simulink model "TP_Automatique_suspension_simulink"  (R2024a)
settings: Solver=ode45  StartTime=0.0  StopTime=10.0  RelTol=1e-3  EnableMultiTasking=on
values from neighbouring files (symbols this model uses):
  R = 24*10^3    (= 24000)    [TP Automatique.m]    (also in TP_Automatique.m = [r_0, r_1, r_2, r_3]; TP_Automatique_2.m = Vecteur_solution(4:7); TP_Automatique_suspension.m = [r_0, r_1, r_2, r_3]; chat.m = theta(1:nr+1).')
  S = [1, sigma_1, sigma_2, sigma_3]    [TP_Automatique.m]    (also in TP_Automatique_2.m = Vecteur_solution(1:3); TP_Automatique_suspension.m = [1, sigma_1, sigma_2, sigma_3, 0]; chat.m = [SA SB]; matlab.mat = [1 40.9 681.8 6077.6 0])
  T = 26.330 * [1 30 300 1000]    [TP_Automatique.m]    (also in TP_Automatique_2.m; TP_Automatique_suspension.m; chat.m = T(end-nb:end))
  U_0 = R*I_0    (= 15570018.9474)    [TP Automatique.m]    (also in TP_Automatique.m = R*I_0; TP_Automatique_2.m = R*I_0; TP_Automatique_suspension.m = R*I_0; chat.m = R*I_0)
  V = poly([-1 , -1, -1, -1])    [TP_Automatique.m]    (also in TP_Automatique_suspension.m; matlab.mat = [1 4 6 4 1])
  V_0 = -alpha*Z_0    (= -15)    [TP_Automatique.m]    (also in TP_Automatique_2.m; TP_Automatique_suspension.m; chat.m)
undefined symbols (not defined in the file or in its folder): sigbuilder_block
settings Model: Creator=2021-1254  LastModifiedBy=Administrator
settings SolverCC: AlgebraicLoopSolver=TrustRegion
settings DataIOCC: LimitDataPoints=on  SaveFormat=Array  ReturnWorkspaceOutputs=off
settings OptimizationCC: LifeSpan=inf
settings DebuggingCC: UnderspecifiedInitializationDetection=Classic  MergeDetectMultiDrivingBlocksExec=none  SolverPrmCheckMsg=warning  UnconnectedInputMsg=warning  UnconnectedOutputMsg=warning  UnconnectedLineMsg=warning  SFUnexpectedBacktrackingDiag=warning  SFNoUnconditionalDefaultTransitionDiag=warning  SFExecutionAtInitializationDiag=none  ArithmeticOperatorsInVariantConditions=warning
settings HardwareCC: ProdBitPerPointer=32  ProdBitPerSizeT=32  ProdBitPerPtrDiffT=32  ProdLargestAtomicFloat=None  ProdIntDivRoundTo=Undefined  ProdEndianess=Unspecified  ProdWordSize=32  ProdHWDeviceType=32-bit Generic
settings ModelReferenceCC: PropagateSignalLabelsOutOfModel=off
settings SFSimCC: SimUseLocalCustomCode=off  CustomCodeUndefinedFunction=UseInterfaceOnly
settings RTWCC: RTWUseLocalCustomCode=off  GPUComputeCapability=3.5
settings CodeAppCC: StateflowObjectComments=on
settings GRTTargetCC: TargetLangStandard=C89/C90 (ANSI)
settings ConfigComp: CovMetricSettings=dw  CovSaveCumulativeToWorkspaceVar=on  CovSaveSingleToWorkspaceVar=on  CovExternalEMLEnable=off

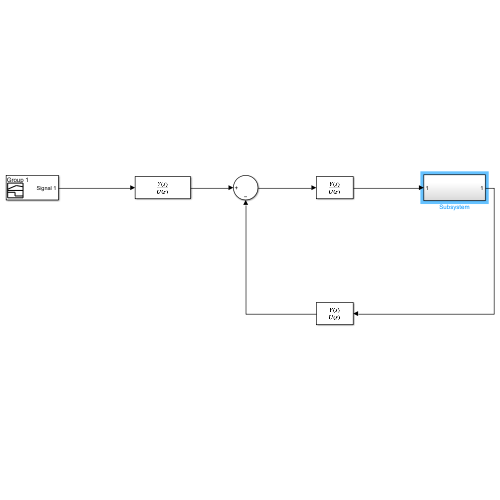
[thumbnail: Simulink's stored preview of the top-level diagram]
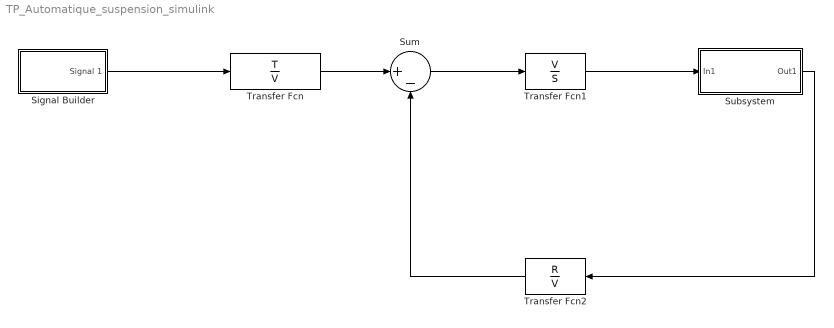
== system TP_Automatique_suspension_simulink ==
  Signal Builder : Subsystem  Tag=STV Subsys  LoadFcn=sigbuilder_block('load');  StartFcn=sigbuilder_block('start');  StopFcn=sigbuilder_block('stop');  ClipboardFcn=sigbuilder_block('clipboard');  mask(Sigbuilder block){tuvar=[0:10]}
      mask help: Simulink:masks:SigbuilderBlock_MD
      mask init:
      | if ~strcmp(get_param(bdroot(gcbh),'SimulationStatus'),'stopped') tuvar = sigbuilder_block('maskInit'); end
      settings: CopyFcn=sigbuilder_block('copy');  DeleteFcn=sigbuilder_block('delete');  ModelCloseFcn=sigbuilder_block('modelClose');  PreSaveFcn=sigbuilder_block('preSave');  PauseFcn=sigbuilder_block('pause');  ContinueFcn=sigbuilder_block('continue');  NameChangeFcn=sigbuilder_block('namechange');  OpenFcn=sigbuilder_block('open',[-284.25 -135 1428 717.75 ]);  CloseFcn=sigbuilder_block('close');
      mask Display: plot(0, 0, 100, 100,[2, 2, 32, 32, 2], [68, 8, 8, 68, 68],[32, 2], [38, 38], [32, 19, 2],[53, 60, 44], [32, 17, 17, 2],[16, 16, 31, 31]);txt = getActiveGroup(gcbh);text(2, 100, txt,'verticalAlignment', 'top');
  Subsystem : Subsystem
  Sum : Sum  Inputs=|+-
  Transfer Fcn : TransferFcn  Numerator=T  Denominator=V
  Transfer Fcn1 : TransferFcn  Numerator=V  Denominator=S
  Transfer Fcn2 : TransferFcn  Numerator=R  Denominator=V
  wires:
  Signal Builder/1(Signal 1) -> Transfer Fcn/1
  Transfer Fcn/1 -> Sum/1
  Transfer Fcn2/1 -> Sum/2
  Transfer Fcn1/1 -> Subsystem/1(In1)
  Sum/1 -> Transfer Fcn1/1
  Subsystem/1(Out1) -> Transfer Fcn2/1

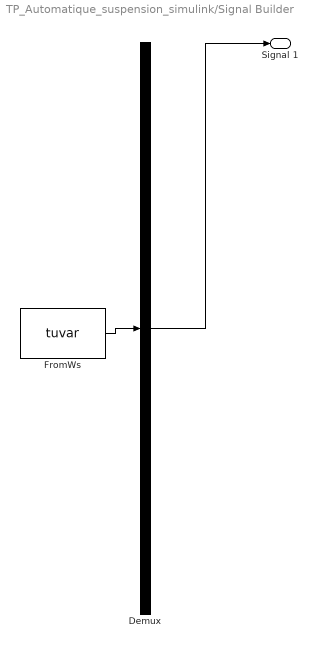
== system TP_Automatique_suspension_simulink/Signal Builder ==
  Demux : Demux  Tag=STV Demux  Outputs=1
      settings: DisplayOption=none
  FromWs : FromWorkspace  Tag=STV FromWs  VariableName=tuvar
      SigBuilderData=|
      | common.afterFinalStr = 'Extrapolate'
      | common.sampleTime = 0
      | dataSet.timeRange = [0 50]
      | dataSet.name = 'Group 1'
      | sbobj.Groups.Name = 'Group 1'
      | sbobj.Groups.Signals.Name = 'Signal 1'
      | sbobj.Groups.Signals.XData = [0 10 10 20 20 30 30 50]
      | sbobj.Groups.Signals.YData = [0 0 -10 -10 -20 -20 0 0]
      | sbobj.Groups.TimeRange = [0 50]
  Signal 1 : Outport  Tag=STV Outport
  wires:
  Demux/1 -> Signal 1/1
  FromWs/1 -> Demux/1

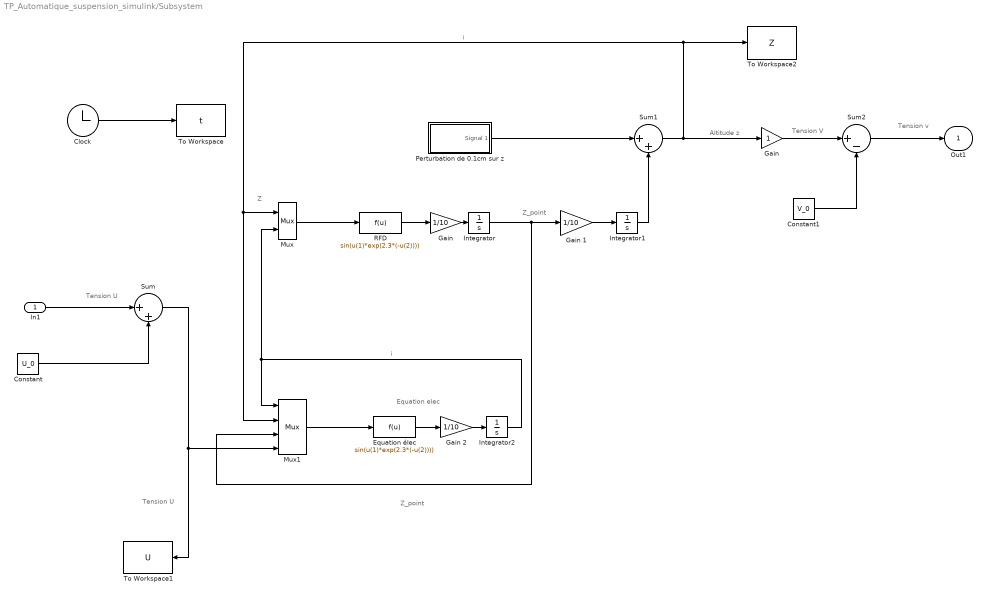
== system TP_Automatique_suspension_simulink/Subsystem ==
  note: Tension v
  note: Tension V
  note: Altitude z
  note: Z
  note: Z_point
  note: Equation elec
  note: Z_point
  note: Tension U
  note: Tension U
  In1 : Inport
  Clock : Clock
  Constant : Constant  Value=U_0
  Constant1 : Constant  Value=V_0
  Equation élec : Fcn  Expr=sin(u(1)*exp(2.3*(-u(2))))
  Gain : Gain
  "Gain " : Gain  Gain=1/10
  "Gain 1 " : Gain  Gain=1/10
  "Gain 2 " : Gain  Gain=1/10
  Integrator : Integrator
  Integrator1 : Integrator
  Integrator2 : Integrator
  Mux : Mux  Inputs=2
  Mux1 : Mux
  Perturbation de 0.1cm sur z : Subsystem  Tag=STV Subsys  LoadFcn=sigbuilder_block('load');  StartFcn=sigbuilder_block('start');  StopFcn=sigbuilder_block('stop');  ClipboardFcn=sigbuilder_block('clipboard');  mask(Sigbuilder block){tuvar=[0:10]}
      mask help: Simulink:masks:SigbuilderBlock_MD
      mask init:
      | if ~strcmp(get_param(bdroot(gcbh),'SimulationStatus'),'stopped') tuvar = sigbuilder_block('maskInit'); end
      settings: CopyFcn=sigbuilder_block('copy');  DeleteFcn=sigbuilder_block('delete');  ModelCloseFcn=sigbuilder_block('modelClose');  PreSaveFcn=sigbuilder_block('preSave');  PauseFcn=sigbuilder_block('pause');  ContinueFcn=sigbuilder_block('continue');  NameChangeFcn=sigbuilder_block('namechange');  OpenFcn=sigbuilder_block('open',[236 5.5 718.5 474.5 ]);  CloseFcn=sigbuilder_block('close');
      mask Display: plot(0, 0, 100, 100,[2, 2, 32, 32, 2], [68, 8, 8, 68, 68],[32, 2], [38, 38], [32, 19, 2],[53, 60, 44], [32, 17, 17, 2],[16, 16, 31, 31]);txt = getActiveGroup(gcbh);text(2, 100, txt,'verticalAlignment', 'top');
  RFD : Fcn  Expr=sin(u(1)*exp(2.3*(-u(2))))
  Sum : Sum  Inputs=|++
  Sum1 : Sum  Inputs=|++
  Sum2 : Sum  Inputs=|+-
  To Workspace : ToWorkspace  VariableName=t  SampleTime=-1
  To Workspace1 : ToWorkspace  VariableName=U  SampleTime=-1
  To Workspace2 : ToWorkspace  VariableName=Z  SampleTime=-1
  Out1 : Outport
  wires:
  In1/1 -> Sum/1
  Constant/1 -> Sum/2
  Clock/1 -> To Workspace/1
  Mux1/1 -> Equation élec/1
  Equation élec/1 -> "Gain 2 "/1
  Sum/1 -> To Workspace1/1, Mux1/4
  Mux/1 -> RFD/1
  RFD/1 -> "Gain "/1
  Perturbation de 0.1cm sur z/1(Signal 1) -> Sum1/1
  Gain/1 -> Sum2/1
  Sum2/1 -> Out1/1
  Integrator1/1 -> Sum1/2
  Integrator/1 -> Mux1/3, "Gain 1 "/1
  Constant1/1 -> Sum2/2
  Sum1/1 -> To Workspace2/1, Mux1/2, Mux/1, Gain/1  "i"
  Integrator2/1 -> Mux1/1, Mux/2  "i"
  "Gain "/1 -> Integrator/1
  "Gain 1 "/1 -> Integrator1/1
  "Gain 2 "/1 -> Integrator2/1

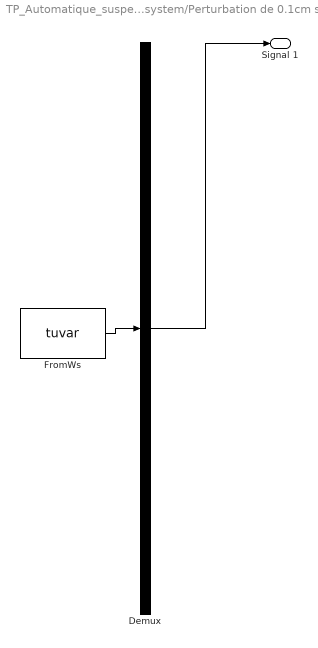
== system TP_Automatique_suspension_simulink/Subsystem/Perturbation de 0.1cm sur z ==
  Demux : Demux  Tag=STV Demux  Outputs=1
      settings: DisplayOption=none
  FromWs : FromWorkspace  Tag=STV FromWs  VariableName=tuvar
      SigBuilderData=|
      | common.afterFinalStr = 'Extrapolate'
      | common.sampleTime = 0
      | dataSet.timeRange = [0 10]
      | dataSet.name = 'Group 1'
      | sbobj.Groups.Name = 'Group 1'
      | sbobj.Groups.Signals.Name = 'Signal 1'
      | sbobj.Groups.Signals.XData = [0 4 4.2 4.22 10]
      | sbobj.Groups.Signals.YData = [0 0 5 0 0]
  Signal 1 : Outport  Tag=STV Outport
  wires:
  Demux/1 -> Signal 1/1
  FromWs/1 -> Demux/1
